simulink model "HEss_conventional_for_comparison"  (R2023a)
settings: Solver=FixedStepAuto  StartTime=0.0  StopTime=2.5  RelTol=1e-3
undefined symbols (not defined in the file): Acid, Lead, sigbuilder_block, Ts
libraries: spsSeriesRLCBranchLib x12, spsMosfetLib x5, spsMeanLib x3, spsPWMGeneratorDCDCLib x3, spsCurrentMeasurementLib x3, spsFirstOrderFilterLib x1, spsBatteryLib x1, spsIdealSwitchLib x1, spsVoltageMeasurementLib x1, spsPVArrayLib x1, spsDiodeLib x1, spsSupercapacitorLib x1
settings Model: Creator=bomma  LastModifiedBy=bomma

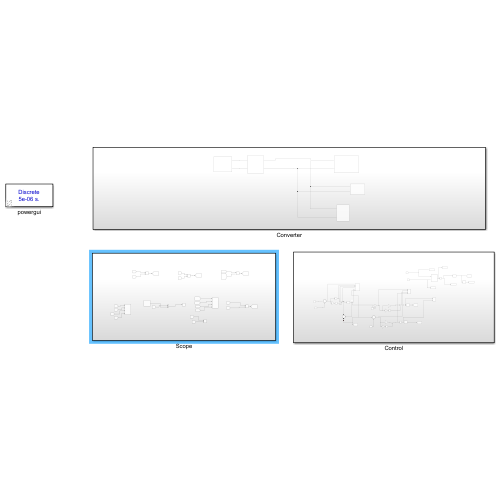
[thumbnail: Simulink's stored preview of the top-level diagram]
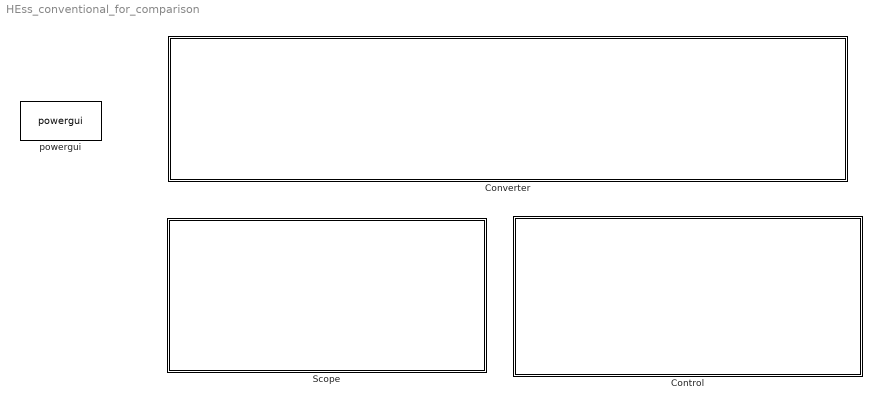
== system HEss_conventional_for_comparison ==
  Control : Subsystem
  Converter : Subsystem
  Scope : Subsystem
  powergui : spspowerguiLib/powergui  Priority=1  SimulationMode=Discrete  SampleTime=Ts  frequency=60  Iterations=50  frequencyindice=0  Pbase=100e6  ErrMax=1e-4  UnitsV=kV  UnitsW=MW  buscounter=0  FunctionMessages=off  echomessages=off  EnableUseOfTLC=off  CurrentSourceSwitches=off  DisableSnubberDevices=off  DisableRonSwitches=off  DisableVfSwitches=off  DisplayEquations=off  AutomaticDiscreteSolvers=off  SolverType=Tustin/Backward Euler (TBE)  Interpol=off  ExternalGateDelay=off  methode=off  Ts=100  x0status=blocks  SPID=on  SwTol=0  HookPort=off  NonlinearTolerance=1e-4  nMaxIteration=100  ContinueOnMaxIteration=off  RestoreLinks=warning  ResistiveCurrentMeasurement=off  Frange=[0:2:500]  Ylog=off  Xlog=on  ShowGrid=off  save=off  variable=ZData  structure=0  ZoomFFT=off  StartTime=0.0  cycles=1  DisplayStyle=1  fundamental=60  FreqAxis=off  MaxFrequency=1000  frequencyindicesteady=1  RmsSteady=1  display=off

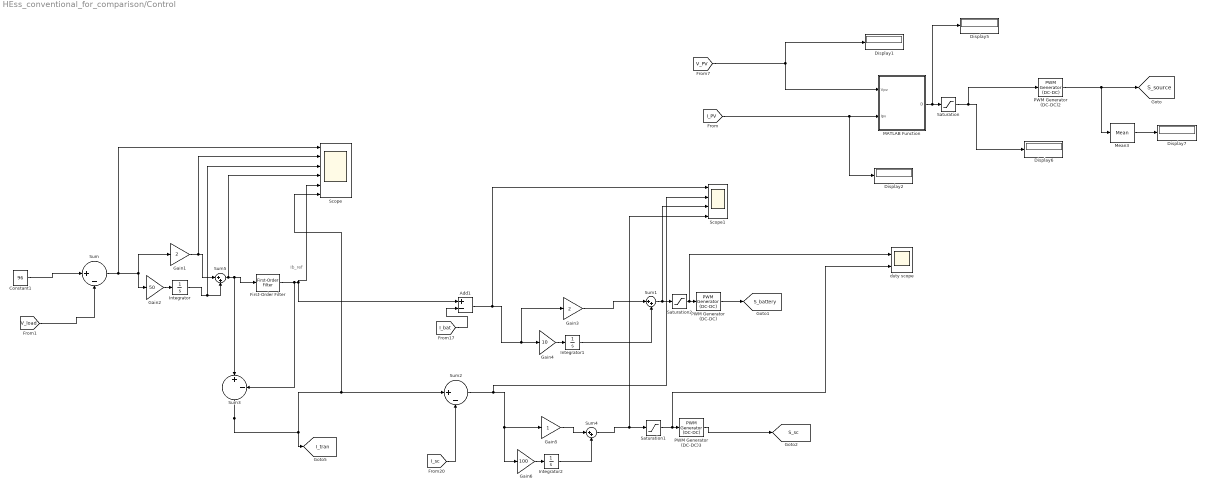
== system HEss_conventional_for_comparison/Control ==
  note: Ib_ref
  Add1 : Sum  Inputs=+-
  Constant1 : Constant  Value=96
  Display{1..2,5..7} (5 alike) : Display
  First-Order Filter : spsFirstOrderFilterLib/First-Order Filter  FilterType=Lowpass  Tc=0.05  Ts=0  Initialize=off  Vac_Init=[0, 0, 60]  Vdc_Init=0  PlotResponse=off  FreqRange="[0,  200,  1]"
  Gain1 : Gain  Gain=2
  Gain2 : Gain  Gain=50
  Gain3 : Gain  Gain=2
  Gain4 : Gain  Gain=10
  Gain5 : Gain
  Gain6 : Gain  Gain=100
  Integrator : Integrator
  Integrator1 : Integrator
  Integrator2 : Integrator
  MATLAB Function : MATLAB Function  TreatAsAtomicUnit=on
  Mean3 : spsMeanLib/Mean  Freq=60  Vinit=0  Ts=0
  PWM Generator (DC-DC) : spsPWMGeneratorDCDCLib/PWM Generator (DC-DC)  Fsw=10e3  Ts=0
  PWM Generator (DC-DC)2 : spsPWMGeneratorDCDCLib/PWM Generator (DC-DC)  Fsw=10e3  Ts=0
  PWM Generator (DC-DC)3 : spsPWMGeneratorDCDCLib/PWM Generator (DC-DC)  Fsw=10e3  Ts=0
  Saturation : Saturate  UpperLimit=0.7  LowerLimit=0.1
  Saturation1 : Saturate  UpperLimit=0.9  LowerLimit=0.1
  Saturation2 : Saturate  UpperLimit=0.9  LowerLimit=0.1
  Scope : Scope  NumInputPorts=6
  Scope1 : Scope  NumInputPorts=4
  Sum : Sum  Inputs=|+-
  Sum1 : Sum  Inputs=|++
  Sum2 : Sum  Inputs=|+-
  Sum3 : Sum  Inputs=|+-
  Sum4 : Sum  Inputs=|++
  Sum5 : Sum  Inputs=|++
  duty scope : Scope  NumInputPorts=2
  tag scope: I_tran=global, S_battery=global, S_sc=global, S_source=global
  wires:
  Sum3/1 -> [I_tran], Scope/6, Sum2/1
  [V_load] -> Sum/2
  First-Order Filter/1 -> Add1/1, Scope/5, Sum3/2
  MATLAB Function/1(D) -> Display5/1, Saturation/1
  Saturation/1 -> PWM Generator (DC-DC)2/1, Display6/1
  PWM Generator (DC-DC)2/1 -> [S_source], Mean3/1
  Mean3/1 -> Display7/1
  Constant1/1 -> Sum/1
  [I_PV] -> Display2/1, MATLAB Function/2(Ipv)
  [V_PV] -> MATLAB Function/1(Vpv), Display1/1
  PWM Generator (DC-DC)/1 -> [S_battery]
  Saturation2/1 -> duty scope/1, PWM Generator (DC-DC)/1
  [I_bat] -> Add1/2
  PWM Generator (DC-DC)3/1 -> [S_sc]
  Saturation1/1 -> duty scope/2, PWM Generator (DC-DC)3/1
  Sum4/1 -> Scope1/4, Saturation1/1
  [I_sc] -> Sum2/2
  Gain1/1 -> Scope/2, Sum5/1
  Integrator/1 -> Scope/3, Sum5/2
  Gain2/1 -> Integrator/1
  Sum/1 -> Scope/1, Gain1/1, Gain2/1
  Sum5/1 -> Scope/4, First-Order Filter/1, Sum3/1
  Add1/1 -> Scope1/1, Gain3/1, Gain4/1
  Gain4/1 -> Integrator1/1
  Sum2/1 -> Scope1/2, Gain6/1, Gain5/1
  Gain6/1 -> Integrator2/1
  Gain3/1 -> Sum1/1
  Integrator1/1 -> Sum1/2
  Sum1/1 -> Scope1/3, Saturation2/1
  Gain5/1 -> Sum4/1
  Integrator2/1 -> Sum4/2

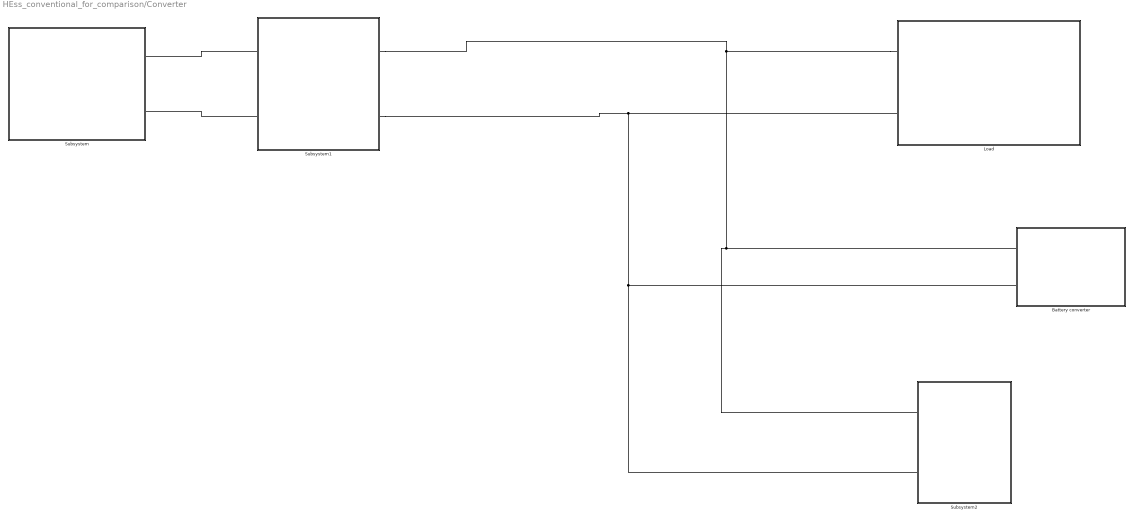
== system HEss_conventional_for_comparison/Converter ==
  Battery converter : Subsystem
  Load : Subsystem
  Subsystem : Subsystem
  Subsystem1 : Subsystem
  Subsystem2 : Subsystem
  connections:
  Subsystem1/LConn1 -- Subsystem/RConn1
  Subsystem1/LConn2 -- Subsystem/RConn2
  Subsystem1/RConn2 -- Subsystem2/LConn2 -- Battery converter/LConn2 -- Load/LConn2
  Load/LConn1 -- Subsystem1/RConn1 -- Subsystem2/LConn1 -- Battery converter/LConn1

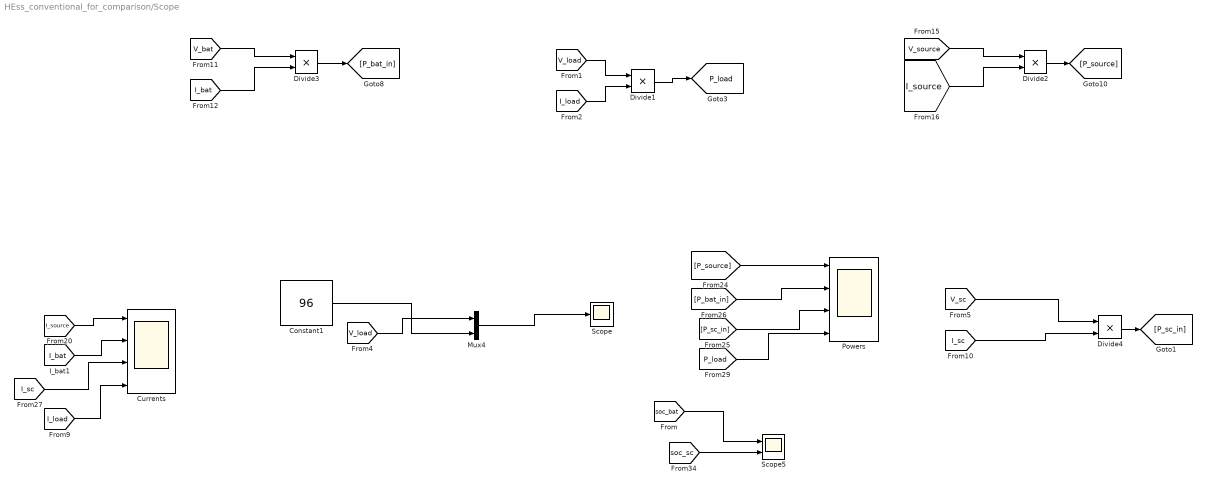
== system HEss_conventional_for_comparison/Scope ==
  Constant1 : Constant  Value=96  SampleTime=Ts
  Currents : Scope  NumInputPorts=4
  Divide{1..4} (4 alike) : Product  Inputs=**
  Mux4 : Mux  Inputs=2
  Powers : Scope  NumInputPorts=4
  Scope : Scope
  Scope5 : Scope  NumInputPorts=2
  tag scope: P_load=global
  wires:
  [V_bat] -> Divide3/1
  [I_bat] -> Divide3/2
  [I_bat] -> Currents/2
  Divide3/1 -> [P_bat_in]
  [V_source] -> Divide2/1
  [P_sc_in] -> Powers/3
  [P_bat_in] -> Powers/2
  [I_load] -> Divide1/2
  [I_source] -> Divide2/2
  Divide2/1 -> [P_source]
  [V_load] -> Divide1/1
  Divide1/1 -> [P_load]
  [P_source] -> Powers/1
  [I_source] -> Currents/1
  Constant1/1 -> Mux4/2
  [V_load] -> Mux4/1
  Mux4/1 -> Scope/1
  Divide4/1 -> [P_sc_in]
  [V_sc] -> Divide4/1
  [I_sc] -> Divide4/2
  [I_load] -> Currents/4
  [I_sc] -> Currents/3
  [P_load] -> Powers/4
  [soc_bat] -> Scope5/1
  [soc_sc] -> Scope5/2

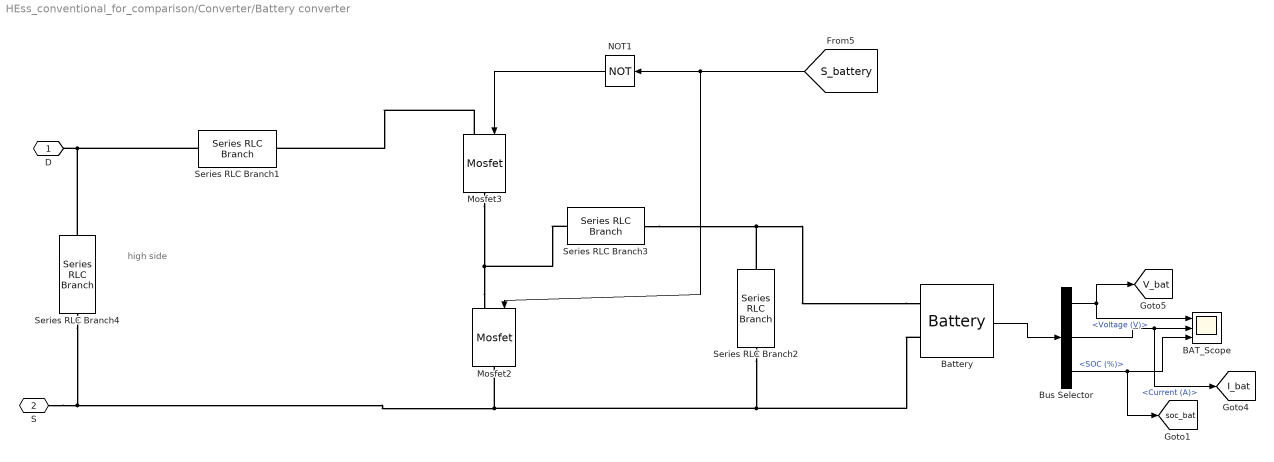
== system HEss_conventional_for_comparison/Converter/Battery converter ==
  note: high side
  BAT_Scope : Scope  NumInputPorts=3
  Battery : spsBatteryLib/Battery  BatType=Lead-Acid  ShowTempParam=off  ThermalPreset=no  ShowAgeParam=off  NomV=48  NomQ=28  SOC=79.997  Batt_Tr=0.1  PresetModel=on  MaxQ=29.1667  MinV=36  FullV=52.2632  Dis_rate=5.6  R=0.017143  Normal_OP=8.6878  expZone="[48.8684    0.0933333]"  current=[6.5 13 32.5]  Units=Time  Tci=20  NomT=20  T2=-30  MaxQ2=4.8  FullV2=7.1  Normal_OP2=5.655  expZone2="[6.58           1]"  Rca=0.6  ti=2000  Dp=0  Neq0=0  Tsim=1e6  Ta1=25  Qeol=5.4*0.9  Reol=0.013333*1.2  Char_age=[2.3478, 3]  Dis_age=[2.3478, 10]  N1=1500  N2=10500  N3=1000  N4=1400  Ta2=45  N5=950
  Bus Selector : BusSelector  OutputSignals=Voltage (V),Current (A),SOC (%)
  Mosfet2 : spsMosfetLib/Mosfet  Ron=0.1  Lon=0  Rd=0.01  Vfd=0  IC=0  Rs=1e5  Cs=inf  Measurements=off
  Mosfet3 : spsMosfetLib/Mosfet  Ron=0.1  Lon=0  Rd=0.01  Vfd=0  IC=0  Rs=1e5  Cs=inf  Measurements=off
  NOT1 : Logic  Operator=NOT  IconShape=distinctive  AllPortsSameDT=off  OutDataTypeStr=boolean
  Series RLC Branch1 : spsSeriesRLCBranchLib/Series RLC Branch  LConnTagsString=__new0  RConnTagsString=__new0  BranchType=L  Resistance=0.01  Inductance=0.75e-3  SetiL0=off  InitialCurrent=0  Capacitance=1e-6  Setx0=off  InitialVoltage=0  Measurements=None
  Series RLC Branch2 : spsSeriesRLCBranchLib/Series RLC Branch  LConnTagsString=__new0  RConnTagsString=__new0  BranchType=RC  Resistance=0.1  Inductance=1e-3  SetiL0=off  InitialCurrent=0  Capacitance=(220e-6)  Setx0=off  InitialVoltage=0  Measurements=None
  Series RLC Branch3 : spsSeriesRLCBranchLib/Series RLC Branch  LConnTagsString=__new0  RConnTagsString=__new0  BranchType=RL  Resistance=0.01  Inductance=2.3e-3  SetiL0=off  InitialCurrent=0  Capacitance=1e-6  Setx0=off  InitialVoltage=0  Measurements=None
  Series RLC Branch4 : spsSeriesRLCBranchLib/Series RLC Branch  LConnTagsString=__new0  RConnTagsString=__new0  BranchType=RC  Resistance=0.1  Inductance=1e-3  SetiL0=off  InitialCurrent=0  Capacitance=(220e-6)  Setx0=off  InitialVoltage=0  Measurements=None
  D : PMIOPort  Side=Left
  S : PMIOPort  Port=2  Side=Left
  tag scope: I_bat=global, V_bat=global, soc_bat=global
  wires:
  Bus Selector/2 -> [I_bat], BAT_Scope/2  "<Current (A)>"
  Bus Selector/1 -> BAT_Scope/1, [V_bat]  "<Voltage (V)>"
  Battery/1 -> Bus Selector/1
  Bus Selector/3 -> BAT_Scope/3, [soc_bat]  "<SOC (%)>"
  NOT1/1 -> Mosfet3/1
  [S_battery] -> Mosfet2/1, NOT1/1
  connections:
  Battery/LConn1 -- Series RLC Branch2/LConn1 -- Series RLC Branch3/RConn1
  Battery/LConn2 -- Series RLC Branch2/RConn1 -- Series RLC Branch4/RConn1 -- S/RConn1 -- Mosfet2/RConn1
  Mosfet2/LConn1 -- Series RLC Branch3/LConn1 -- Mosfet3/RConn1
  Series RLC Branch1/LConn1 -- Series RLC Branch4/LConn1 -- D/RConn1
  Mosfet3/LConn1 -- Series RLC Branch1/RConn1

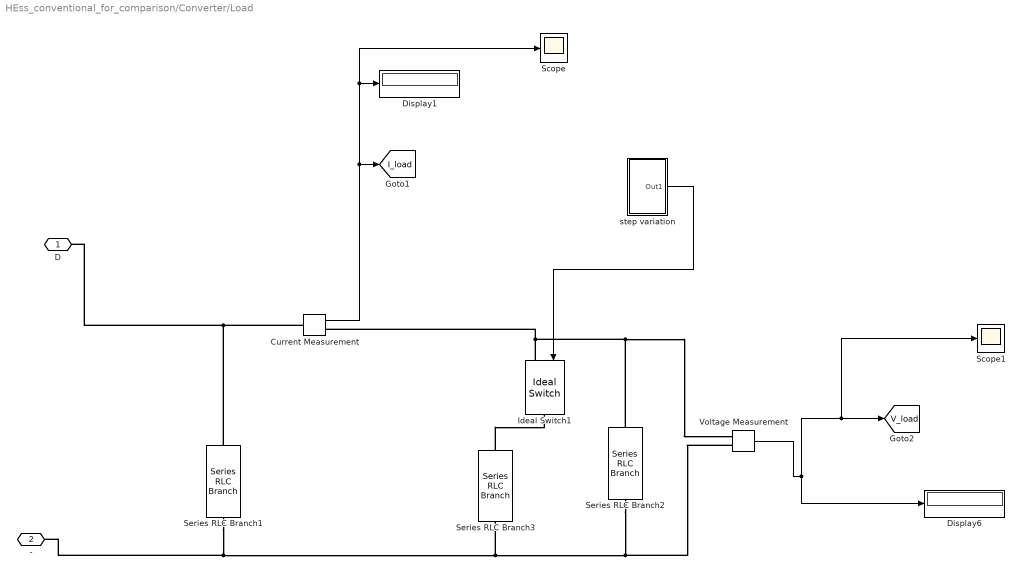
== system HEss_conventional_for_comparison/Converter/Load ==
  Current Measurement : spsCurrentMeasurementLib/Current Measurement  PhasorSimulation=off  OutputType=Complex  PSBequivalent=0
  Display1 : Display
  Display6 : Display
  Ideal Switch1 : spsIdealSwitchLib/Ideal Switch  Ron=0.001  Lon=0  IC=0  Rs=1e5  Cs=inf  Measurements=off
  Scope : Scope
  Scope1 : Scope
  Series RLC Branch1 : spsSeriesRLCBranchLib/Series RLC Branch  LConnTagsString=__new0  RConnTagsString=__new0  BranchType=C  Resistance=0.1  Inductance=1e-3  SetiL0=off  InitialCurrent=0  Capacitance=430e-6  Setx0=off  InitialVoltage=24  Measurements=None
  Series RLC Branch2 : spsSeriesRLCBranchLib/Series RLC Branch  LConnTagsString=__new0  RConnTagsString=__new0  BranchType=R  Resistance=48  Inductance=1e-3  SetiL0=off  InitialCurrent=0  Capacitance=1e-6  Setx0=off  InitialVoltage=0  Measurements=None
  Series RLC Branch3 : spsSeriesRLCBranchLib/Series RLC Branch  LConnTagsString=__new0  RConnTagsString=__new0  BranchType=R  Resistance=50  Inductance=1e-3  SetiL0=off  InitialCurrent=0  Capacitance=1e-6  Setx0=off  InitialVoltage=0  Measurements=None
  Voltage Measurement : spsVoltageMeasurementLib/Voltage Measurement  PhasorSimulation=off  OutputType=Complex  PSBequivalent=0
  step variation : Subsystem
  D : PMIOPort  Side=Left
  - : PMIOPort  Port=2  Side=Left
  tag scope: I_load=global, V_load=global
  wires:
  Voltage Measurement/1 -> Display6/1, Scope1/1, [V_load]
  Current Measurement/1 -> Scope/1, Display1/1, [I_load]
  step variation/1(Out1) -> Ideal Switch1/1
  connections:
  Series RLC Branch2/LConn1 -- Voltage Measurement/LConn1 -- Current Measurement/RConn1 -- Ideal Switch1/LConn1
  -/RConn1 -- Series RLC Branch3/RConn1 -- Series RLC Branch2/RConn1 -- Voltage Measurement/LConn2 -- Series RLC Branch1/RConn1
  Current Measurement/LConn1 -- Series RLC Branch1/LConn1 -- D/RConn1
  Series RLC Branch3/LConn1 -- Ideal Switch1/RConn1

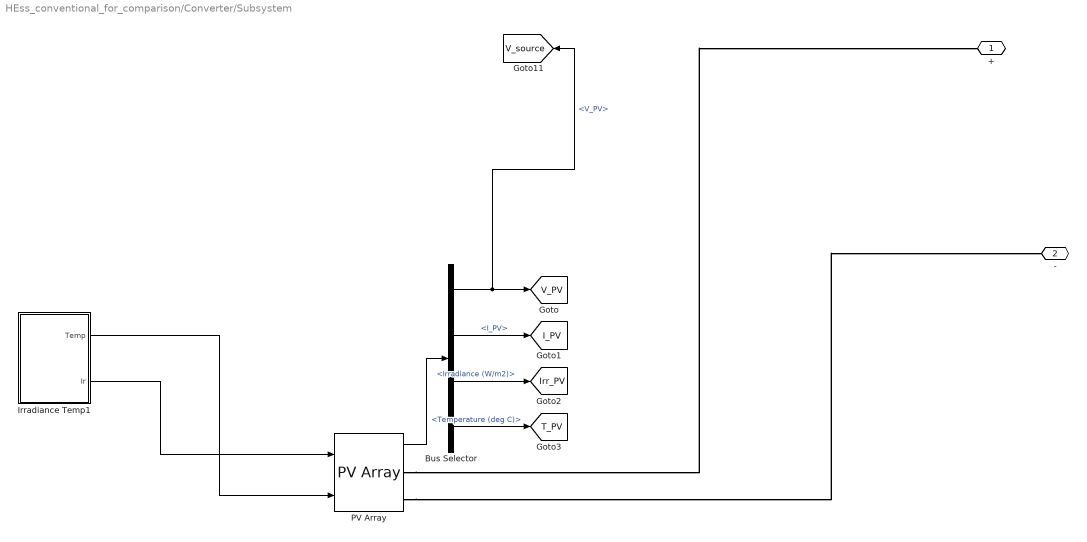
== system HEss_conventional_for_comparison/Converter/Subsystem ==
  Bus Selector : BusSelector  OutputSignals=V_PV,I_PV,Irradiance (W/m2),Temperature (deg C)
  Irradiance Temp1 : Subsystem  Tag=STV Subsys  LoadFcn=sigbuilder_block('load');  StartFcn=sigbuilder_block('start');  StopFcn=sigbuilder_block('stop');  ClipboardFcn=sigbuilder_block('clipboard');  mask(Sigbuilder block){tuvar=[0:10]}
      mask help: Sigbuilder GUI
      mask init:
      | if ~strcmp(get_param(bdroot(gcbh),'SimulationStatus'),'stopped') tuvar = sigbuilder_block('maskInit'); end
      settings: CopyFcn=sigbuilder_block('copy');  DeleteFcn=sigbuilder_block('delete');  ModelCloseFcn=sigbuilder_block('modelClose');  PreSaveFcn=sigbuilder_block('preSave');  PauseFcn=sigbuilder_block('pause')  ContinueFcn=sigbuilder_block('continue')  NameChangeFcn=sigbuilder_block('namechange');  OpenFcn=sigbuilder_block('open',[5.5 36 949 472 ]);  CloseFcn=sigbuilder_block('close');
      mask Display: plot(0, 0, 100, 100,[2, 2, 32, 32, 2], [68, 8, 8, 68, 68],[32, 2], [38, 38], [32, 19, 2],[53, 60, 44], [32, 17, 17, 2],[16, 16, 31, 31]);txt = getActiveGroup(gcbh);text(2, 100, txt,'verticalAlignment', 'top');
  PV Array : spsPVArrayLib/PV Array  Npar=1  Nser=2  PlotType=array @ 25 deg.C & specified irradiances  S_vec="[ 1000 800 500  250 ]"  Temp_C_vec="[0 25 50  ]"  ModuleName=A10Green Technology A10J-M60-220  PlotWhenSelected=on  Pm=219.876  Ncell=60  Voc=36.06  Isc=7.95  Vm=30.12  Im=7.3  beta_Voc_pc=-0.3624  alpha_Isc_pc=0.054805  beta_Voc=-0.13068  alpha_Isc=0.004357  IL=7.9642  I0=2.8692e-10  nI=0.97455  Rsh=106.1817  Rs=0.18964  RobustModel=off  RobustCellTemperature=313.3991  BAL=on  Tc=Tc  Tfilter=5e-5
  + : PMIOPort  Side=Right
  - : PMIOPort  Port=2  Side=Right
  tag scope: I_PV=global, Irr_PV=global, T_PV=global, V_PV=global, V_source=global
  wires:
  PV Array/1 -> Bus Selector/1
  Bus Selector/4 -> [T_PV]  "<Temperature (deg C)>"
  Bus Selector/1 -> [V_source], [V_PV]  "<V_PV>"
  Irradiance Temp1/1(Temp) -> PV Array/2
  Bus Selector/3 -> [Irr_PV]  "<Irradiance (W/m2)>"
  Bus Selector/2 -> [I_PV]  "<I_PV>"
  Irradiance Temp1/2(Ir) -> PV Array/1
  connections:
  PV Array/RConn2 -- -/RConn1
  PV Array/RConn1 -- +/RConn1

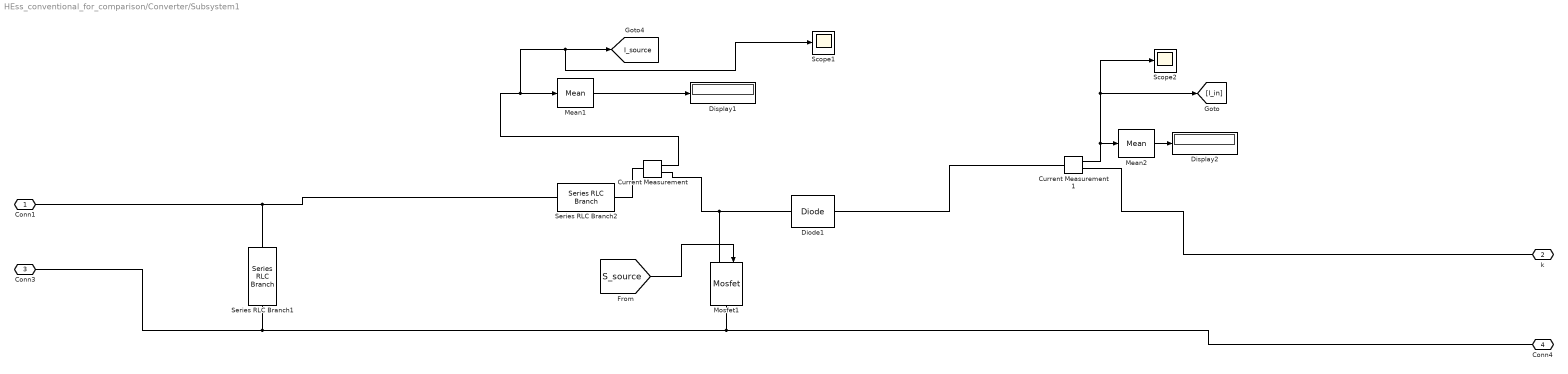
== system HEss_conventional_for_comparison/Converter/Subsystem1 ==
  Current Measurement : spsCurrentMeasurementLib/Current Measurement  PhasorSimulation=off  OutputType=Complex  PSBequivalent=0
  Current Measurement1 : spsCurrentMeasurementLib/Current Measurement  PhasorSimulation=off  OutputType=Complex  PSBequivalent=0
  Diode1 : spsDiodeLib/Diode  Ron=0.001  Lon=0  Vf=0.8  IC=0  UseSnubber=0  Rs=500  Cs=250e-9  Measurements=off
  Display1 : Display
  Display2 : Display
  Mean1 : spsMeanLib/Mean  Freq=60  Vinit=0  Ts=0
  Mean2 : spsMeanLib/Mean  Freq=60  Vinit=0  Ts=0
  Mosfet1 : spsMosfetLib/Mosfet  Ron=0.1  Lon=0  Rd=0.01  Vfd=0  IC=0  Rs=1e5  Cs=inf  Measurements=off
  Scope1 : Scope
  Scope2 : Scope
  Series RLC Branch1 : spsSeriesRLCBranchLib/Series RLC Branch  LConnTagsString=__new0  RConnTagsString=__new0  BranchType=RC  Resistance=0.01  Inductance=1e-3  SetiL0=off  InitialCurrent=0  Capacitance=2.2e-6  Setx0=off  InitialVoltage=0  Measurements=None
  Series RLC Branch2 : spsSeriesRLCBranchLib/Series RLC Branch  LConnTagsString=__new0  RConnTagsString=__new0  BranchType=RL  Resistance=0.1  Inductance=3.1e-3  SetiL0=off  InitialCurrent=0  Capacitance=10e-6  Setx0=off  InitialVoltage=0  Measurements=None
  Conn1 : PMIOPort  Side=Left
  k : PMIOPort  Port=2  Side=Right
  Conn3 : PMIOPort  Port=3  Side=Left
  Conn4 : PMIOPort  Port=4  Side=Right
  tag scope: I_source=global
  wires:
  Current Measurement/1 -> Scope1/1, [I_source], Mean1/1
  [S_source] -> Mosfet1/1
  Mean1/1 -> Display1/1
  Mean2/1 -> Display2/1
  Current Measurement1/1 -> Mean2/1, [I_in], Scope2/1
  connections:
  Current Measurement1/RConn1 -- k/RConn1
  Series RLC Branch2/LConn1 -- Conn1/RConn1 -- Series RLC Branch1/LConn1
  Series RLC Branch2/RConn1 -- Current Measurement/LConn1
  Mosfet1/LConn1 -- Diode1/LConn1 -- Current Measurement/RConn1
  Series RLC Branch1/RConn1 -- Conn3/RConn1 -- Conn4/RConn1 -- Mosfet1/RConn1
  Current Measurement1/LConn1 -- Diode1/RConn1

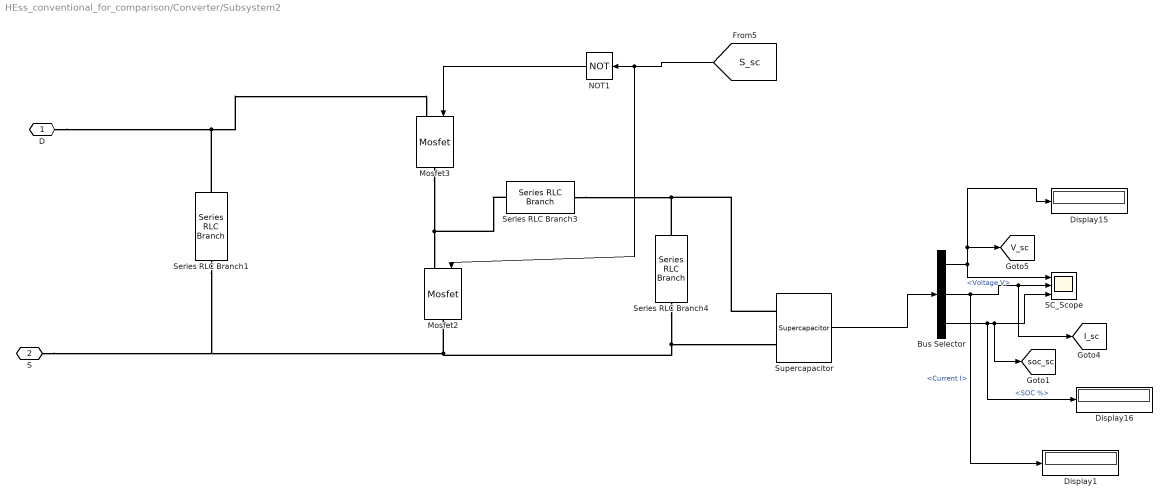
== system HEss_conventional_for_comparison/Converter/Subsystem2 ==
  Bus Selector : BusSelector  OutputSignals=Voltage V,Current I,SOC %
  Display1 : Display
  Display15 : Display
  Display16 : Display
  Mosfet2 : spsMosfetLib/Mosfet  Ron=0.1  Lon=0  Rd=0.01  Vfd=0  IC=0  Rs=1e5  Cs=inf  Measurements=off
  Mosfet3 : spsMosfetLib/Mosfet  Ron=0.1  Lon=0  Rd=0.01  Vfd=0  IC=0  Rs=1e5  Cs=inf  Measurements=off
  NOT1 : Logic  Operator=NOT  IconShape=distinctive  AllPortsSameDT=off  OutDataTypeStr=boolean
  SC_Scope : Scope  NumInputPorts=3
  Series RLC Branch1 : spsSeriesRLCBranchLib/Series RLC Branch  LConnTagsString=__new0  RConnTagsString=__new0  BranchType=RC  Resistance=0.1  Inductance=1e-3  SetiL0=off  InitialCurrent=0  Capacitance=(220e-6)  Setx0=off  InitialVoltage=0  Measurements=None
  Series RLC Branch3 : spsSeriesRLCBranchLib/Series RLC Branch  LConnTagsString=__new0  RConnTagsString=__new0  BranchType=L  Resistance=0.01  Inductance=2.3e-3  SetiL0=off  InitialCurrent=0  Capacitance=1e-6  Setx0=off  InitialVoltage=0  Measurements=None
  Series RLC Branch4 : spsSeriesRLCBranchLib/Series RLC Branch  LConnTagsString=__new0  RConnTagsString=__new0  BranchType=RC  Resistance=0.1  Inductance=1e-3  SetiL0=off  InitialCurrent=0  Capacitance=(220e-6)  Setx0=off  InitialVoltage=0  Measurements=None
  Supercapacitor : spsSupercapacitorLib/Supercapacitor  C=19.3  Rdc=8.9e-3  Voltage=48  Ns=1  Np=1  Vinit=47  Temp=25  PresetModel=off  EstParam=off  Nc=1  r=1e-9  epsilon=6.0208e-10  Ich=10  Vstern="[0.161  2.7  7.8]"  Self_dis=on  Ioc=10  Vself="[48  47.8  47.06  44.65]"  demandeplot=off  I="[10  20 100  500]"  Units=sec  Vmax=0  If=0  deltaV=0  alpha=0  sec=0
      settings: LibrarySourceBlock=sps_lib/Sources/Supercapacitor
  D : PMIOPort  Side=Left
  S : PMIOPort  Port=2  Side=Left
  tag scope: I_sc=global, V_sc=global, soc_sc=global
  wires:
  Supercapacitor/1 -> Bus Selector/1
  Bus Selector/2 -> Display1/1, [I_sc], SC_Scope/2  "<Current I>"
  [S_sc] -> Mosfet2/1, NOT1/1
  Bus Selector/1 -> SC_Scope/1, Display15/1, [V_sc]  "<Voltage V>"
  Bus Selector/3 -> Display16/1, SC_Scope/3, [soc_sc]  "<SOC %>"
  NOT1/1 -> Mosfet3/1
  connections:
  Series RLC Branch3/RConn1 -- Supercapacitor/LConn1 -- Series RLC Branch4/LConn1
  Series RLC Branch4/RConn1 -- Series RLC Branch1/RConn1 -- S/RConn1 -- Mosfet2/RConn1 -- Supercapacitor/LConn2
  Mosfet3/RConn1 -- Mosfet2/LConn1 -- Series RLC Branch3/LConn1
  D/RConn1 -- Mosfet3/LConn1 -- Series RLC Branch1/LConn1

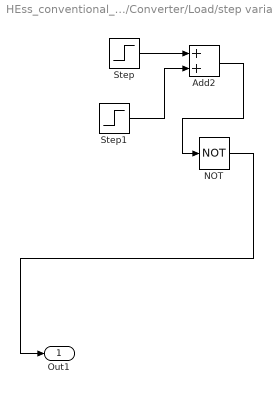
== system HEss_conventional_for_comparison/Converter/Load/step variation ==
  Add2 : Sum
  NOT : Logic  Operator=NOT  IconShape=distinctive  AllPortsSameDT=off  OutDataTypeStr=boolean
  Step : Step  Time=2  SampleTime=0
  Step1 : Step  Time=1.5  Before=1  After=0  SampleTime=0
  Out1 : Outport
  wires:
  Add2/1 -> NOT/1
  NOT/1 -> Out1/1
  Step/1 -> Add2/1
  Step1/1 -> Add2/2

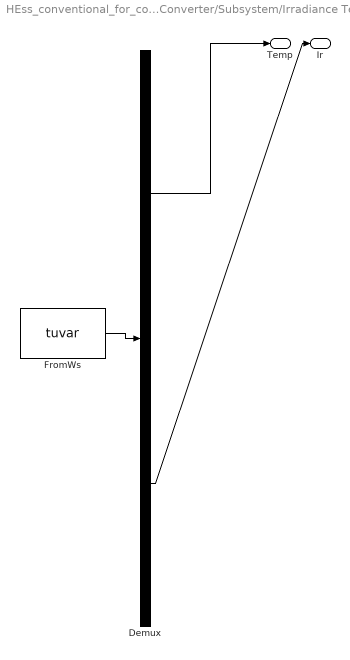
== system HEss_conventional_for_comparison/Converter/Subsystem/Irradiance Temp1 ==
  Demux : Demux  Tag=STV Demux  Outputs=2
      settings: DisplayOption=none
  FromWs : FromWorkspace  Tag=STV FromWs  VariableName=tuvar
      SigBuilderData=|
      | common.afterFinalStr = 'Extrapolate'
      | common.sampleTime = '0'
      | dataSet(1).timeRange = [0 2]
      | dataSet(1).name = 'Constant Irradiance'
      | dataSet(2).timeRange = [0 4]
      | dataSet(2).name = 'Step Irradiance'
      | dataSet(3).timeRange = [0 2.5]
      | dataSet(3).name = 'Ramp-up/down Irradiance'
      | sbobj.Groups(1).Name = 'Constant Irradiance'
      | sbobj.Groups(1).Signals(1).Name = 'Temp'
      | sbobj.Groups(1).Signals(1).XData = [0 1 1 2]
      | sbobj.Groups(1).Signals(1).YData = [0 0 1 1]
      | sbobj.Groups(1).Signals(2).Name = 'Ir'
      | sbobj.Groups(1).Signals(2).XData = [0 0.8 0.8 1.2 1.2 2]
      | sbobj.Groups(1).Signals(2).YData = [0 0 1 1 0 0]
      | sbobj.Groups(1).TimeRange = [0 2]
      | sbobj.Groups(2).Name = 'Step Irradiance'
      | sbobj.Groups(2).Signals(1).Name = 'Temp'
      | sbobj.Groups(2).Signals(1).XData = [0 1 1 4]
      | sbobj.Groups(2).Signals(1).YData = [0 0 1 1]
      | sbobj.Groups(2).Signals(2).Name = 'Ir'
      | sbobj.Groups(2).Signals(2).XData = [0 0.8 0.8 1.2 1.2 4]
      | sbobj.Groups(2).Signals(2).YData = [0 0 1 1 0 0]
      | sbobj.Groups(2).TimeRange = [0 4]
      | sbobj.Groups(3).Name = 'Ramp-up/down Irradiance'
      | sbobj.Groups(3).Signals(1).Name = 'Temp'
      | sbobj.Groups(3).Signals(1).XData = [0 2.5]
      | sbobj.Groups(3).Signals(1).YData = [25 25]
      | sbobj.Groups(3).Signals(2).Name = 'Ir'
      | sbobj.Groups(3).Signals(2).XData = [0 0.5 0.5 1 1 2.5]
      | sbobj.Groups(3).Signals(2).YData = [500 500 1000 1000 500 500]
      | sbobj.Groups(3).TimeRange = [0 2.5]
  Temp : Outport  Tag=STV Outport
  Ir : Outport  Tag=STV Outport  Port=2
  wires:
  FromWs/1 -> Demux/1
  Demux/1 -> Temp/1
  Demux/2 -> Ir/1

== matlab function HEss_conventional_for_comparison/Control/MATLAB Function ==
  settings: updateMethod=DISCRETE  sampleTime=1e-4
  data: Vpv input; D output; Ipv input
function D = PandO(Vpv,Ipv)

persistent Dold Pold Vold


if isempty(Dold)
    Dold = 0.35;
    Vold = 17;
    Pold = 120;
end


deltaD = 0.001;

Ppv = Vpv*Ipv;

if (Ppv-Pold) ~= 0
    if (Ppv-Pold) > 0
        if (Vpv-Vold) > 0
            D = Dold - deltaD;
        else
            D = Dold + deltaD;
        end
    else
        if (Vpv-Vold) > 0
            D = Dold + deltaD;
        else
            D = Dold - deltaD;
        end        
    end
else
    D = Dold;
end

Dold = D;
Vold = Vpv;
Pold = Ppv;
